simulink model "ZeroCrossingModel"  (R2014a)
settings: Solver=ode45  StartTime=0.0  StopTime=10.0  RelTol=1e-3
settings Model: Creator=lgw  LastModifiedBy=李广文

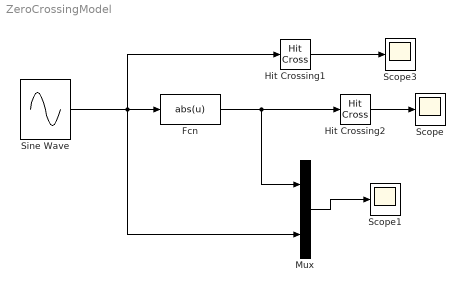
== system ZeroCrossingModel ==
  Fcn : Fcn  Expr=abs(u)
  Hit Crossing1 : HitCross
  Hit Crossing2 : HitCross  HitCrossingOffset=0.5
  Mux : Mux  Inputs=2
  Scope : Scope
  Scope1 : Scope
  Scope3 : Scope
      settings: SaveName=ScopeData3
  Sine Wave : Sin  SampleTime=0
  wires:
  Mux/1 -> Scope1/1
  Fcn/1 -> Hit Crossing2/1, Mux/1
  Sine Wave/1 -> Mux/2, Hit Crossing1/1, Fcn/1
  Hit Crossing1/1 -> Scope3/1
  Hit Crossing2/1 -> Scope/1
